simulink model "Simulink_P4"  (R2025a)
settings: Solver=VariableStepAuto  StartTime=0.0  StopTime=10.0  MaxStep=0.05  RelTol=1e-3
InitFcn:
  | m = 10;
  | k = 100;

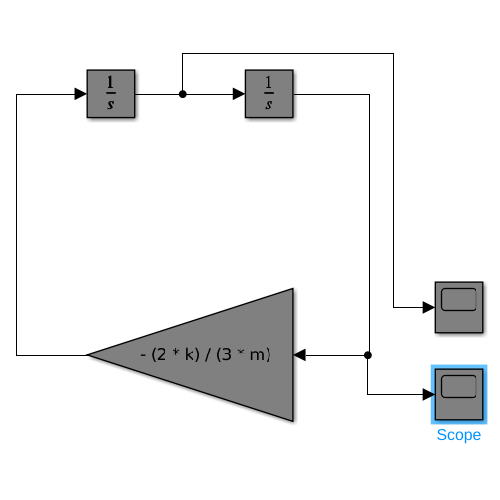
[thumbnail: Simulink's stored preview of the top-level diagram]
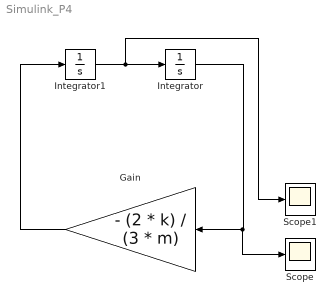
== system Simulink_P4 ==
  Gain : Gain  Gain=- (2 * k) / (3 * m)
  Integrator : Integrator
  Integrator1 : Integrator  InitialCondition=2
  Scope : Scope
      settings: ActiveDisplayYMinimum=-0.9680836375674049  ActiveDisplayYMaximum=0.96809083072350088
  Scope1 : Scope
      settings: ActiveDisplayYMinimum=-2.4999915139392379  ActiveDisplayYMaximum=2.4999990571043598
  wires:
  Integrator1/1 -> Integrator/1, Scope1/1
  Gain/1 -> Integrator1/1
  Integrator/1 -> Scope/1, Gain/1
